simulink model "sampleModel301"  (R2021b)
settings: Solver=VariableStepAuto  StartTime=0.0  StopTime=10.0  RelTol=1e-3
libraries: simulink x15, slpidlib x3
settings Model: Creator=user  LastModifiedBy=user

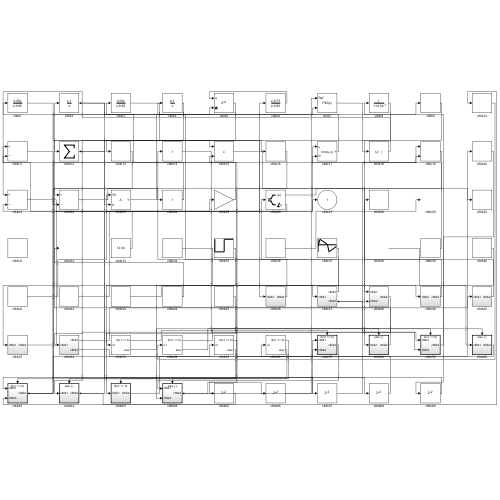
[thumbnail: Simulink's stored preview of the top-level diagram]
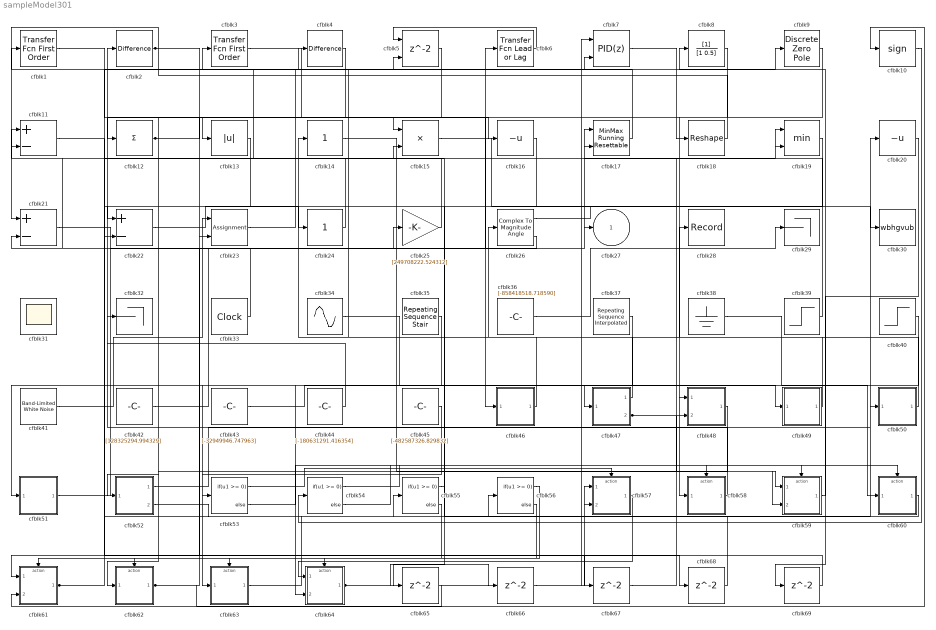
== system sampleModel301 ==
  cfblk1 : simulink/Discrete/Transfer Fcn First Order  PoleZ=0.95  ICPrevOutput=0.0  DoSatur=off
  cfblk10 : Signum
  cfblk11 : Sum  Inputs=+-
  cfblk12 : Sum  Inputs=+
  cfblk13 : Abs
  cfblk14 : simulink/Math Operations/Slider Gain  gain=1  low=0  high=2
  cfblk15 : Product  Inputs=**
  cfblk16 : UnaryMinus
  cfblk17 : simulink/Math Operations/MinMax Running Resettable  Function=min  vinit=0.0
  cfblk18 : Reshape
  cfblk19 : MinMax  Inputs=2
  cfblk2 : simulink/Discrete/Difference  ICPrevInput=0.0  OutMin=[]  OutMax=[]  OutDataTypeStr=Inherit: Inherit via back propagation  OutDataType=fixdt(1, 16)  OutScaling=2^-10  DoSatur=off
  cfblk20 : UnaryMinus
  cfblk21 : Sum  Inputs=+-
  cfblk22 : Sum  Inputs=+-
  cfblk23 : Assignment  DiagnosticForDimensions=Warning  IndexOptions=Index vector (dialog)  Indices=1  OutputSizes=1
  cfblk24 : simulink/Math Operations/Slider Gain  gain=1  low=0  high=2
  cfblk25 : Gain  Gain=[249708222.524312]
  cfblk26 : ComplexToMagnitudeAngle
  cfblk28 : Record  FileSettingsInternal="{\"entries\":[{\"content\":{\"excelSettings\":{\"content\":{},\"type\":\"Streamout.ExcelSettings\"}},\"type\":\"Streamout.FileSettingStorage\",\"uuid\":\"fc3e83d0-d56b-4c83-b2a5-80e353ecfa04\"}],\"packageUris\":[\"http://schema.mathworks.com/mf0/streamout_blocks/R2020a\"],\"version\":\"1.0\"}"  SignalsInternal="{\"entries\":[{\"content\":{\"signals\":[{\"content\":{\"blockPath\":[\"sampleModel301/cfblk28\"],\"channel\":[],\"dimensions\":[1],\"domain\":\"sampleModel301/cfblk28\",\"lineColor\":\"#0072bd\",\"plots\":[1],\"port\":1,\"sid\":[\"\"],\"signalID\":12922,\"signalName\":\"cfblk49\"},\"type\":\"RecordBlkView.Signal\",\"uuid\":\"28842435-4abb-4854-9952-0d3e1e0a5988\"}]},\"type\":\"RecordBlkView.InputSignals\",\"uuid\":\"907c0131-cf25-44c8-b84d-6c3f6b91576e\"}],\"packageUris\":[\"http://schema.mathworks.com/mf0/streamout_blocks/R2020a\"],\"version\":\"1.0\"}"  VisualizationBindings="{\"sparklinesplugin\":{\"info\":[{\"bindingParametersList\":[],\"subplotID\":1}]}}"
  cfblk29 : Terminator
  cfblk3 : simulink/Discrete/Transfer Fcn First Order  PoleZ=0.95  ICPrevOutput=0.0  DoSatur=off
  cfblk30 : ToWorkspace  VariableName=wbhgvub  SaveFormat=Timeseries  SampleTime=-1
  cfblk31 : Scope
      settings: Floating=on
  cfblk32 : Terminator
  cfblk33 : DigitalClock
  cfblk34 : Sin  Amplitude=[15370521.272923]  Bias=[-395037117.474888]  SampleTime=0
  cfblk35 : simulink/Sources/Repeating Sequence Stair  OutValues=[-750649913.169033, -673104103.156418]  tsamp=-1  OutMin=[]  OutMax=[]  OutDataTypeStr=double  OutputDataTypeScalingMode=double  OutDataType=fixdt(0,8)  ConRadixGroup=Best Precision: Vector-wise  OutScaling=2^-12
  cfblk36 : Constant  Value=[-858418518.718590]  SampleTime=1
  cfblk37 : simulink/Sources/Repeating Sequence Interpolated  OutValues=[-162004117.785946, 546396170.857113, 46021324.132391, -691416578.945760, -166491336.279565]  TimeValues=[0 0.1 0.5 0.6 1].'  LookUpMeth=Use Input Above  tsamp=0.01  OutMin=[]  OutMax=[]  OutDataTypeStr=double  OutputDataTypeScalingMode=double  OutDataType=fixdt(0,8)  OutScaling=2^-10
  cfblk38 : Ground
  cfblk39 : Step  Time=[14.000000]  Before=[69064811.287218]  After=[727866125.826064]  SampleTime=0
  cfblk4 : simulink/Discrete/Difference  ICPrevInput=0.0  OutMin=[]  OutMax=[]  OutDataTypeStr=Inherit: Inherit via back propagation  OutDataType=fixdt(1, 16)  OutScaling=2^-10  DoSatur=off
  cfblk40 : Step  Time=[42.000000]  Before=[-690044896.559738]  After=[-801015617.864337]  SampleTime=0
  cfblk41 : simulink/Sources/Band-Limited White Noise  Cov=[2192988932.714114]  Ts=0.1  seed=[4336989221.000000]
  cfblk42 : Constant  Value=[128325294.994329]  SampleTime=1
  cfblk43 : Constant  Value=[-32949946.747963]  SampleTime=1
  cfblk44 : Constant  Value=[-180631291.416354]  SampleTime=1
  cfblk45 : Constant  Value=[-482587326.829832]  SampleTime=1
  cfblk46 : Subsystem
  cfblk47 : Subsystem
  cfblk48 : Subsystem
  cfblk49 : Subsystem
  cfblk5 : Delay  ShowEnablePort=on  SampleTime=1
      settings: InputPortMap=u0,e6
  cfblk50 : Subsystem
  cfblk51 : Subsystem
  cfblk52 : Subsystem
  cfblk{53..56} (4 alike) : If  IfExpression=u1 >= 0  SampleTime=1
  cfblk57 : Subsystem  TreatAsAtomicUnit=on
  cfblk58 : Subsystem  TreatAsAtomicUnit=on
  cfblk59 : Subsystem  TreatAsAtomicUnit=on
  cfblk6 : simulink/Discrete/Transfer Fcn Lead or Lag  PoleZ=0.95  ZeroZ=0.75  ICPrevOutput=0.0  ICPrevInput=0.0  DoSatur=off
      settings: SourceProductBaseCode=SL
  cfblk60 : Subsystem  TreatAsAtomicUnit=on
  cfblk61 : Subsystem  TreatAsAtomicUnit=on
  cfblk62 : Subsystem  TreatAsAtomicUnit=on
  cfblk63 : Subsystem  TreatAsAtomicUnit=on
  cfblk64 : Subsystem  TreatAsAtomicUnit=on
  cfblk{65..69} (5 alike) : Delay  SampleTime=1
  cfblk7 : slpidlib/PID Controller (2DOF)  Controller=PID  Form=Parallel  TimeDomain=Discrete-time  UseExternalTs=off  SampleTime=1  IntegratorMethod=Forward Euler  FilterMethod=Forward Euler  ControllerParametersSource=internal  P=1  I=1  D=0  UseFilter=on  N=100  b=1  c=1  TunerSelectOption=Transfer Function Based (PID Tuner App)  InitialConditionSource=internal  InitialConditionForIntegrator=0  InitialConditionForFilter=0  DifferentiatorICPrevScaledInput=0  ExternalReset=none  TrackingMode=off  Kt=1  LimitOutput=off  SatLimitsSource=internal  UpperSaturationLimit=inf  LowerSaturationLimit=-inf  LinearizeAsGain=off  AntiWindupMode=none  Kb=1  POutMin=[]  POutMax=[]  IOutMin=[]  IOutMax=[]  DOutMin=[]  DOutMax=[]  NOutMin=[]  NOutMax=[]  bOutMin=[]  bOutMax=[]  cOutMin=[]  cOutMax=[]  SumOutMin=[]  SumOutMax=[]  SaturationOutMin=[]  SaturationOutMax=[]  PParamMin=[]  PParamMax=[]  IParamMin=[]  IParamMax=[]  DParamMin=[]  DParamMax=[]  NParamMin=[]  NParamMax=[]  bParamMin=[]  bParamMax=[]  cParamMin=[]  cParamMax=[]  KbParamMin=[]  KbParamMax=[]  KtParamMin=[]  KtParamMax=[]  KbOutMin=[]  KbOutMax=[]  KtOutMin=[]  KtOutMax=[]  IntegratorOutMin=[]  IntegratorOutMax=[]  FilterOutMin=[]  FilterOutMax=[]  SumI1OutMin=[]  SumI1OutMax=[]  SumI2OutMin=[]  SumI2OutMax=[]  SumI3OutMin=[]  SumI3OutMax=[]  SumI4OutMin=[]  SumI4OutMax=[]  SumDOutMin=[]  SumDOutMax=[]  Sum1OutMin=[]  Sum1OutMax=[]  Sum2OutMin=[]  Sum2OutMax=[]  Sum3OutMin=[]  Sum3OutMax=[]  DifferentiatorOutMin=[]  DifferentiatorOutMax=[]  FilterDiffOutCoefMin=[]  FilterDiffOutCoefMax=[]  ReciprocalOutMin=[]  ReciprocalOutMax=[]  SumDenOutMin=[]  SumDenOutMax=[]  SumNumOutMin=[]  SumNumOutMax=[]  DivideOutMin=[]  DivideOutMax=[]  UdiffTsProdOutMin=[]  UdiffTsProdOutMax=[]  NTsProdOutMin=[]  NTsProdOutMax=[]  UintegralTsProdOutMin=[]  UintegralTsProdOutMax=[]  UngainTsProdOutMin=[]  UngainTsProdOutMax=[]  IntegratorContinuousStateAttributes=''  IntegratorStateMustResolveToSignalObject=off  IntegratorRTWStateStorageClass=Auto  FilterContinuousStateAttributes=''  FilterStateMustResolveToSignalObject=off  FilterRTWStateStorageClass=Auto  ParallelPVariant=InternalParameters  IdealPVariant=Disabled  IVariant=InternalParameters  DVariant=InternalParameters  bVariant=InternalParameters  cVariant=InternalParameters  IntegratorVariant=Discrete  SatVariant=Disabled  AWVariant=Passthrough  PCopyVariant=Disabled  TRVariant=Disabled  FdbkBlocksVariant=Forward  IdealPFdbkVariant=Disabled  SatFdbkVariant=Disabled  DerivativeFilterVariant=ForwardEulerFilter  NVariant=InternalParameters  NCopyVariant=Disabled  FilterICVariant=InternalICsFilter  IntegratorICVariant=InternalICs  ExternalResetVariant=Disabled  TRSumVariant=Passthrough  SumFdbkVariant=Disabled  SumVariant=Sum_PID  TsampFilterVariant=InternalTs  TsampNgainVariant=Passthrough  TsampIntegralVariant=Passthrough  ExternalSaturationOutDataTypeStr=Inherit: Same as second input
      settings: SourceProductBaseCode=SL
  cfblk8 : DiscreteFilter  SampleTime=1
  cfblk9 : DiscreteZeroPole  Poles=[0 0.5]  Gain=1
  cfblk27 : Outport
  wires:
  cfblk39/1 -> cfblk17/1
  cfblk46/1(cfblk2) -> cfblk14/1
  cfblk22/1 -> cfblk24/1
  cfblk59/1(cfblk2) -> cfblk8/1
  cfblk44/1 -> cfblk2/1
  cfblk18/1 -> cfblk21/1
  cfblk60/1(cfblk2) -> cfblk56/1
  cfblk19/1 -> cfblk22/1
  cfblk24/1 -> cfblk11/1
  cfblk8/1 -> cfblk12/1
  cfblk10/1 -> cfblk54/1
  cfblk50/1(cfblk2) -> cfblk26/1
  cfblk40/1 -> cfblk51/1(cfblk1)
  cfblk3/1 -> cfblk46/1(cfblk1)
  cfblk41/1 -> cfblk23/1
  cfblk9/1 -> cfblk58/1(cfblk1)
  cfblk35/1 -> cfblk63/1(cfblk1)
  cfblk51/1(cfblk2) -> cfblk17/2
  cfblk34/1 -> cfblk47/1(cfblk1)
  cfblk63/1(cfblk2) -> cfblk20/1
  cfblk1/1 -> cfblk15/1
  cfblk5/1 -> cfblk52/1(cfblk1)
  cfblk15/1 -> cfblk48/1(cfblk1)
  cfblk7/1 -> cfblk18/1
  cfblk42/1 -> cfblk6/1
  cfblk2/1 -> cfblk23/2, cfblk5/2
  cfblk64/1(cfblk2) -> cfblk7/1, cfblk66/1
  cfblk52/1(cfblk2) -> cfblk50/1(cfblk1)
  cfblk62/1(cfblk2) -> cfblk10/1, cfblk25/1
  cfblk33/1 -> cfblk11/2
  cfblk45/1 -> cfblk53/1
  cfblk21/1 -> cfblk27/1
  cfblk52/2(cfblk3) -> cfblk55/1
  cfblk48/1(cfblk2) -> cfblk62/1(cfblk1)
  cfblk38/1 -> cfblk60/1(cfblk1)
  cfblk4/1 -> cfblk13/1
  cfblk49/1(cfblk2) -> cfblk28/1
  cfblk23/1 -> cfblk9/1
  cfblk13/1 -> cfblk22/2
  cfblk17/1 -> cfblk1/1
  cfblk6/1 -> cfblk5/1
  cfblk25/1 -> cfblk3/1
  cfblk58/1(cfblk2) -> cfblk32/1
  cfblk57/1(cfblk2) -> cfblk64/1(cfblk1)
  cfblk12/1 -> cfblk16/1, cfblk68/1
  cfblk26/1 -> cfblk30/1
  cfblk61/1(cfblk2) -> cfblk57/1(cfblk1), cfblk19/2, cfblk7/2
  cfblk43/1 -> cfblk49/1(cfblk1)
  cfblk36/1 -> cfblk29/1
  cfblk26/2 -> cfblk21/2
  cfblk47/1(cfblk2) -> cfblk4/1
  cfblk37/1 -> cfblk64/2(cfblk4)
  cfblk14/1 -> cfblk59/1(cfblk1)
  cfblk47/2(cfblk5) -> cfblk19/1, cfblk59/2(cfblk3)
  cfblk53/1 -> cfblk57/Action
  cfblk53/2 -> cfblk58/Action
  cfblk54/1 -> cfblk59/Action
  cfblk54/2 -> cfblk60/Action
  cfblk55/1 -> cfblk61/Action
  cfblk55/2 -> cfblk62/Action
  cfblk56/1 -> cfblk63/Action
  cfblk56/2 -> cfblk64/Action
  cfblk16/1 -> cfblk65/1
  cfblk65/1 -> cfblk61/2(cfblk3)
  cfblk66/1 -> cfblk57/2(cfblk4)
  cfblk11/1 -> cfblk67/1
  cfblk67/1 -> cfblk48/2(cfblk4)
  cfblk68/1 -> cfblk15/2
  cfblk20/1 -> cfblk69/1
  cfblk69/1 -> cfblk61/1(cfblk1)

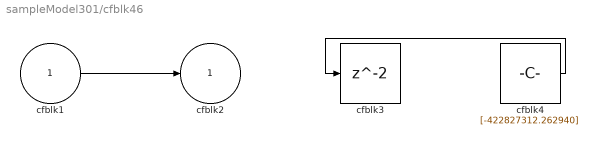
== system sampleModel301/cfblk46 ==
  cfblk1 : Inport
  cfblk3 : Delay  SampleTime=1
  cfblk4 : Constant  Value=[-422827312.262940]  SampleTime=1
  cfblk2 : Outport
  wires:
  cfblk1/1 -> cfblk2/1
  cfblk4/1 -> cfblk3/1

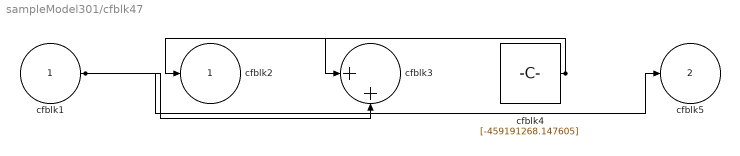
== system sampleModel301/cfblk47 ==
  cfblk1 : Inport
  cfblk3 : Sum  Inputs=|++
  cfblk4 : Constant  Value=[-459191268.147605]  SampleTime=1
  cfblk2 : Outport
  cfblk5 : Outport  Port=2
  wires:
  cfblk4/1 -> cfblk2/1, cfblk3/1
  cfblk1/1 -> cfblk5/1, cfblk3/2

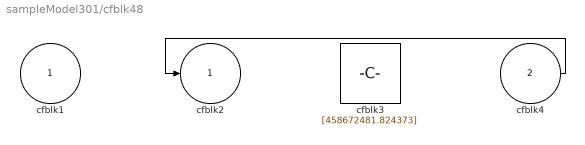
== system sampleModel301/cfblk48 ==
  cfblk1 : Inport
  cfblk4 : Inport  Port=2
  cfblk3 : Constant  Value=[458672481.824373]  SampleTime=1
  cfblk2 : Outport
  wires:
  cfblk4/1 -> cfblk2/1

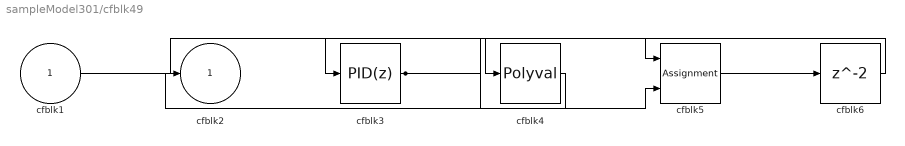
== system sampleModel301/cfblk49 ==
  cfblk1 : Inport
  cfblk3 : slpidlib/PID Controller  Controller=PID  Form=Parallel  TimeDomain=Discrete-time  UseExternalTs=off  SampleTime=1  IntegratorMethod=Forward Euler  FilterMethod=Forward Euler  ControllerParametersSource=internal  P=1  I=1  D=0  UseFilter=on  N=100  TunerSelectOption=Transfer Function Based (PID Tuner App)  InitialConditionSource=internal  InitialConditionForIntegrator=0  InitialConditionForFilter=0  DifferentiatorICPrevScaledInput=0  ExternalReset=none  TrackingMode=off  Kt=1  LimitOutput=off  SatLimitsSource=internal  UpperSaturationLimit=inf  LowerSaturationLimit=-inf  LinearizeAsGain=off  AntiWindupMode=none  Kb=1  POutMin=[]  POutMax=[]  IOutMin=[]  IOutMax=[]  DOutMin=[]  DOutMax=[]  NOutMin=[]  NOutMax=[]  SumOutMin=[]  SumOutMax=[]  SaturationOutMin=[]  SaturationOutMax=[]  PParamMin=[]  PParamMax=[]  IParamMin=[]  IParamMax=[]  DParamMin=[]  DParamMax=[]  NParamMin=[]  NParamMax=[]  KbParamMin=[]  KbParamMax=[]  KtParamMin=[]  KtParamMax=[]  KbOutMin=[]  KbOutMax=[]  KtOutMin=[]  KtOutMax=[]  IntegratorOutMin=[]  IntegratorOutMax=[]  FilterOutMin=[]  FilterOutMax=[]  SumI1OutMin=[]  SumI1OutMax=[]  SumI2OutMin=[]  SumI2OutMax=[]  SumI3OutMin=[]  SumI3OutMax=[]  SumI4OutMin=[]  SumI4OutMax=[]  SumDOutMin=[]  SumDOutMax=[]  DifferentiatorOutMin=[]  DifferentiatorOutMax=[]  FilterDiffOutCoefMin=[]  FilterDiffOutCoefMax=[]  ReciprocalOutMin=[]  ReciprocalOutMax=[]  SumDenOutMin=[]  SumDenOutMax=[]  SumNumOutMin=[]  SumNumOutMax=[]  DivideOutMin=[]  DivideOutMax=[]  UdiffTsProdOutMin=[]  UdiffTsProdOutMax=[]  NTsProdOutMin=[]  NTsProdOutMax=[]  UintegralTsProdOutMin=[]  UintegralTsProdOutMax=[]  UngainTsProdOutMin=[]  UngainTsProdOutMax=[]  IntegratorContinuousStateAttributes=''  IntegratorStateMustResolveToSignalObject=off  IntegratorRTWStateStorageClass=Auto  FilterContinuousStateAttributes=''  FilterStateMustResolveToSignalObject=off  FilterRTWStateStorageClass=Auto  ParallelPVariant=InternalParameters  IdealPVariant=Disabled  IVariant=InternalParameters  DVariant=InternalParameters  IntegratorVariant=Discrete  SatVariant=Disabled  AWVariant=Passthrough  PCopyVariant=Disabled  TRVariant=Disabled  FdbkBlocksVariant=Forward  IdealPFdbkVariant=Disabled  SatFdbkVariant=Disabled  DerivativeFilterVariant=ForwardEulerFilter  NVariant=InternalParameters  NCopyVariant=Disabled  FilterICVariant=InternalICsFilter  IntegratorICVariant=InternalICs  ExternalResetVariant=Disabled  TRSumVariant=Passthrough  SumFdbkVariant=Disabled  SumVariant=Sum_PID  TsampFilterVariant=InternalTs  TsampNgainVariant=Passthrough  TsampIntegralVariant=Passthrough  ExternalSaturationOutDataTypeStr=Inherit: Same as second input
  cfblk4 : Polyval  Coefs=[ +2.081618890e-019, -1.441693666e-014, +4.719686976e-010, -8.536869453e-006, +1.621573104e-001, -8.087801117e+001 ]
  cfblk5 : Assignment  DiagnosticForDimensions=Warning  IndexOptions=Index vector (dialog)  Indices=1  OutputSizes=1
  cfblk6 : Delay  SampleTime=1
  cfblk2 : Outport
  wires:
  cfblk1/1 -> cfblk4/1
  cfblk4/1 -> cfblk2/1
  cfblk3/1 -> cfblk5/1, cfblk5/2
  cfblk5/1 -> cfblk6/1
  cfblk6/1 -> cfblk3/1

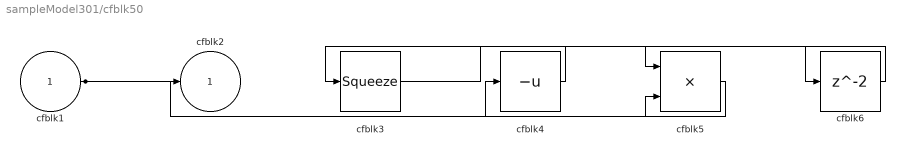
== system sampleModel301/cfblk50 ==
  cfblk1 : Inport
  cfblk3 : Squeeze
  cfblk4 : UnaryMinus
  cfblk5 : Product
  cfblk6 : Delay  SampleTime=1
  cfblk2 : Outport
  wires:
  cfblk4/1 -> cfblk3/1
  cfblk5/1 -> cfblk4/1
  cfblk1/1 -> cfblk5/2, cfblk2/1
  cfblk3/1 -> cfblk6/1
  cfblk6/1 -> cfblk5/1

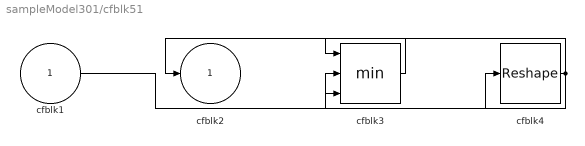
== system sampleModel301/cfblk51 ==
  cfblk1 : Inport
  cfblk3 : MinMax  Inputs=3
  cfblk4 : Reshape
  cfblk2 : Outport
  wires:
  cfblk3/1 -> cfblk2/1
  cfblk1/1 -> cfblk4/1
  cfblk4/1 -> cfblk3/1, cfblk3/2, cfblk3/3

== system sampleModel301/cfblk52 ==
  cfblk1 : Inport
  cfblk2 : Outport
  cfblk3 : Outport  Port=2
  wires:
  cfblk1/1 -> cfblk2/1, cfblk3/1

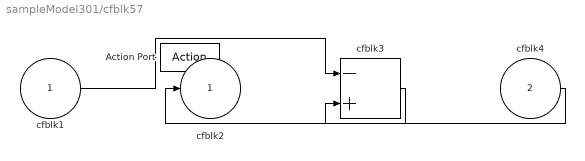
== system sampleModel301/cfblk57 ==
  cfblk1 : Inport
  cfblk4 : Inport  Port=2
  Action Port : ActionPort  ActionPortLabel=if(u1 >= 0)
  cfblk3 : Sum  Inputs=-+
  cfblk2 : Outport
  wires:
  cfblk3/1 -> cfblk2/1
  cfblk1/1 -> cfblk3/1
  cfblk4/1 -> cfblk3/2

== system sampleModel301/cfblk58 ==
  cfblk1 : Inport
  Action Port : ActionPort  ActionPortLabel=else
  cfblk3 : simulink/Discrete/Transfer Fcn First Order  PoleZ=0.95  ICPrevOutput=0.0  DoSatur=off
  cfblk2 : Outport
  wires:
  cfblk1/1 -> cfblk3/1
  cfblk3/1 -> cfblk2/1

== system sampleModel301/cfblk59 ==
  cfblk1 : Inport
  cfblk3 : Inport  Port=2
  Action Port : ActionPort  ActionPortLabel=if(u1 >= 0)
  cfblk2 : Outport
  wires:
  cfblk1/1 -> cfblk2/1

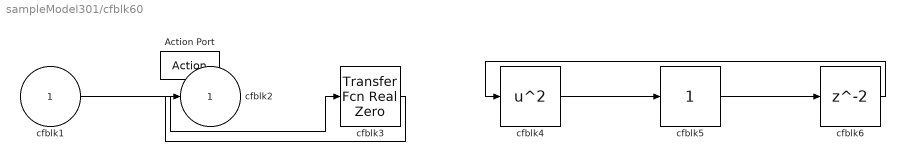
== system sampleModel301/cfblk60 ==
  cfblk1 : Inport
  Action Port : ActionPort  ActionPortLabel=else
  cfblk3 : simulink/Discrete/Transfer Fcn Real Zero  ZeroZ=0.75  ICPrevInput=0.0  DoSatur=off
      settings: SourceProductBaseCode=SL
  cfblk4 : Math  Operator=square  SaturateOnIntegerOverflow=on
  cfblk5 : simulink/Math Operations/Slider Gain  gain=1  low=0  high=2
  cfblk6 : Delay
  cfblk2 : Outport
  wires:
  cfblk4/1 -> cfblk5/1
  cfblk1/1 -> cfblk3/1
  cfblk3/1 -> cfblk2/1
  cfblk5/1 -> cfblk6/1
  cfblk6/1 -> cfblk4/1

== system sampleModel301/cfblk61 ==
  cfblk1 : Inport
  cfblk3 : Inport  Port=2
  Action Port : ActionPort  ActionPortLabel=if(u1 >= 0)
  cfblk2 : Outport
  wires:
  cfblk3/1 -> cfblk2/1

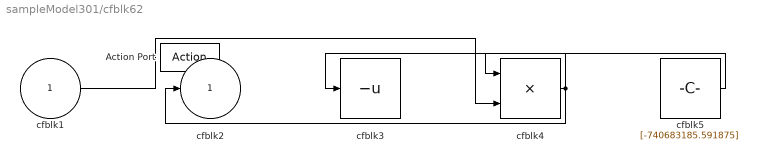
== system sampleModel301/cfblk62 ==
  cfblk1 : Inport
  Action Port : ActionPort  ActionPortLabel=else
  cfblk3 : UnaryMinus
  cfblk4 : Product  Inputs=**
  cfblk5 : Constant  Value=[-740683185.591875]  SampleTime=1
  cfblk2 : Outport
  wires:
  cfblk4/1 -> cfblk2/1, cfblk3/1
  cfblk5/1 -> cfblk4/1
  cfblk1/1 -> cfblk4/2

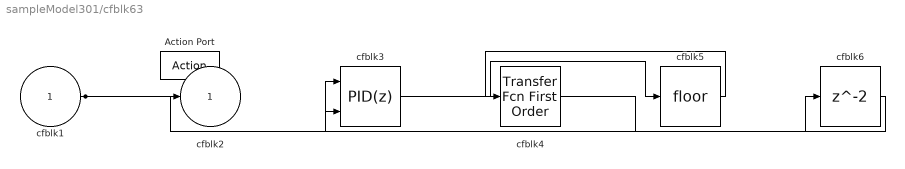
== system sampleModel301/cfblk63 ==
  cfblk1 : Inport
  Action Port : ActionPort  ActionPortLabel=if(u1 >= 0)
  cfblk3 : slpidlib/PID Controller (2DOF)  Controller=PID  Form=Parallel  TimeDomain=Discrete-time  UseExternalTs=off  SampleTime=-1  IntegratorMethod=Forward Euler  FilterMethod=Forward Euler  ControllerParametersSource=internal  P=1  I=1  D=0  UseFilter=on  N=100  b=1  c=1  TunerSelectOption=Transfer Function Based (PID Tuner App)  InitialConditionSource=internal  InitialConditionForIntegrator=0  InitialConditionForFilter=0  DifferentiatorICPrevScaledInput=0  ExternalReset=none  TrackingMode=off  Kt=1  LimitOutput=off  SatLimitsSource=internal  UpperSaturationLimit=inf  LowerSaturationLimit=-inf  LinearizeAsGain=off  AntiWindupMode=none  Kb=1  POutMin=[]  POutMax=[]  IOutMin=[]  IOutMax=[]  DOutMin=[]  DOutMax=[]  NOutMin=[]  NOutMax=[]  bOutMin=[]  bOutMax=[]  cOutMin=[]  cOutMax=[]  SumOutMin=[]  SumOutMax=[]  SaturationOutMin=[]  SaturationOutMax=[]  PParamMin=[]  PParamMax=[]  IParamMin=[]  IParamMax=[]  DParamMin=[]  DParamMax=[]  NParamMin=[]  NParamMax=[]  bParamMin=[]  bParamMax=[]  cParamMin=[]  cParamMax=[]  KbParamMin=[]  KbParamMax=[]  KtParamMin=[]  KtParamMax=[]  KbOutMin=[]  KbOutMax=[]  KtOutMin=[]  KtOutMax=[]  IntegratorOutMin=[]  IntegratorOutMax=[]  FilterOutMin=[]  FilterOutMax=[]  SumI1OutMin=[]  SumI1OutMax=[]  SumI2OutMin=[]  SumI2OutMax=[]  SumI3OutMin=[]  SumI3OutMax=[]  SumI4OutMin=[]  SumI4OutMax=[]  SumDOutMin=[]  SumDOutMax=[]  Sum1OutMin=[]  Sum1OutMax=[]  Sum2OutMin=[]  Sum2OutMax=[]  Sum3OutMin=[]  Sum3OutMax=[]  DifferentiatorOutMin=[]  DifferentiatorOutMax=[]  FilterDiffOutCoefMin=[]  FilterDiffOutCoefMax=[]  ReciprocalOutMin=[]  ReciprocalOutMax=[]  SumDenOutMin=[]  SumDenOutMax=[]  SumNumOutMin=[]  SumNumOutMax=[]  DivideOutMin=[]  DivideOutMax=[]  UdiffTsProdOutMin=[]  UdiffTsProdOutMax=[]  NTsProdOutMin=[]  NTsProdOutMax=[]  UintegralTsProdOutMin=[]  UintegralTsProdOutMax=[]  UngainTsProdOutMin=[]  UngainTsProdOutMax=[]  IntegratorContinuousStateAttributes=''  IntegratorStateMustResolveToSignalObject=off  IntegratorRTWStateStorageClass=Auto  FilterContinuousStateAttributes=''  FilterStateMustResolveToSignalObject=off  FilterRTWStateStorageClass=Auto  ParallelPVariant=InternalParameters  IdealPVariant=Disabled  IVariant=InternalParameters  DVariant=InternalParameters  bVariant=InternalParameters  cVariant=InternalParameters  IntegratorVariant=Discrete  SatVariant=Disabled  AWVariant=Passthrough  PCopyVariant=Disabled  TRVariant=Disabled  FdbkBlocksVariant=Forward  IdealPFdbkVariant=Disabled  SatFdbkVariant=Disabled  DerivativeFilterVariant=ForwardEulerFilter  NVariant=InternalParameters  NCopyVariant=Disabled  FilterICVariant=InternalICsFilter  IntegratorICVariant=InternalICs  ExternalResetVariant=Disabled  TRSumVariant=Passthrough  SumFdbkVariant=Disabled  SumVariant=Sum_PID  TsampFilterVariant=InternalTs  TsampNgainVariant=Passthrough  TsampIntegralVariant=Passthrough  ExternalSaturationOutDataTypeStr=Inherit: Same as second input
      settings: SourceProductBaseCode=SL
  cfblk4 : simulink/Discrete/Transfer Fcn First Order  PoleZ=0.95  ICPrevOutput=0.0  DoSatur=off
  cfblk5 : Rounding
  cfblk6 : Delay
  cfblk2 : Outport
  wires:
  cfblk3/1 -> cfblk5/1
  cfblk1/1 -> cfblk3/1, cfblk2/1
  cfblk5/1 -> cfblk4/1
  cfblk4/1 -> cfblk6/1
  cfblk6/1 -> cfblk3/2

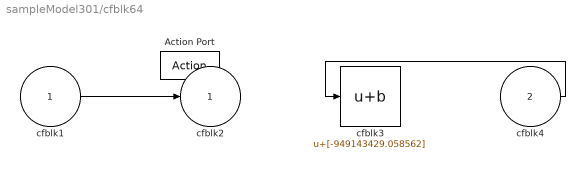
== system sampleModel301/cfblk64 ==
  cfblk1 : Inport
  cfblk4 : Inport  Port=2
  Action Port : ActionPort  ActionPortLabel=else
  cfblk3 : Bias  Bias=[-949143429.058562]
  cfblk2 : Outport
  wires:
  cfblk4/1 -> cfblk3/1
  cfblk1/1 -> cfblk2/1
